simulink model "Motor_Pos_LTI_cl"  (Simulink 7.5)
settings: Solver=VariableStepDiscrete  StartTime=0.0  StopTime=0.1  RelTol=1e-3
libraries: discretizing x1
settings Model: Creator=maen  LastModifiedBy=Rick

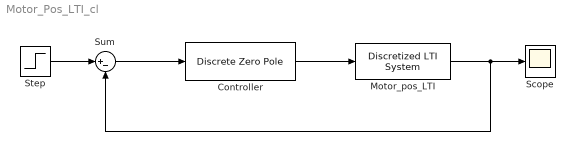
== system Motor_Pos_LTI_cl ==
  Controller : DiscreteZeroPole  Zeros=[0.95 0.80 0.80]  Poles=[-0.98 0.6 1]  Gain=800  SampleTime=0.001
  Motor_pos_LTI : discretizing/Discretized LTI System  SystemSampleTime=-1  sysc=ss(A, B, C, D)  cic=[0]  SampleTime=0.00100000000000000002  method=zoh  Wc=0
  Scope : Scope
      settings: YMin=1.0025  YMax=1.04
  Step : Step  Time=0  SampleTime=0.001
  Sum : Sum  Inputs=|+-  OutDataType=fixdt(1, 16)  OutScaling=2^0  SampleTime=0.001
  wires:
  Controller/1 -> Motor_pos_LTI/1
  Step/1 -> Sum/1
  Sum/1 -> Controller/1
  Motor_pos_LTI/1 -> Scope/1, Sum/2
